simulink library "Kitchen_Lib"  (R2023a)
settings: Solver=VariableStepAuto  StartTime=0.0  StopTime=10.0  RelTol=1e-3  EnableMultiTasking=on
undefined symbols (not defined in the file): Kitc_BusTyp_P, Kitc_BusTypSkyr_C, Kitc_ColrLedColrls_C, Kitc_ColrLedGrn_C, Kitc_ColrLedRed_C, Kitc_ColrLedYlw_C, Kitc_StDgnWtrTank_C, Kitc_StElecPlugScktOffByClmp50_P, Kitc_StsDlyBlink_C, Kitc_StsErrBlink_C, Kitc_StsFctAcvn_P, Kitc_StsInfoBlink_C, Kitc_StsKitchnOffAutoIgOff_P, Kitc_StsKitchnOffBySwt_P, Kitc_StsKitchnOffDoorLockd_P, Kitc_StsKitchnOffIgOff_P, Kitc_StsKitchnOffUv_P, Kitc_StsKitchnOnBySwt_P, Kitc_StsKitchnOnNVM_P, Kitc_StsLedOff_C, Kitc_StsLedOn_C, Kitc_StsLrgCnsAcv_P, Kitc_StTrfrAnSwtInstd_P, Kitc_StTrfrSwtInstd_P, Kitc_TiKitcRefgtrOffDly_P, Kitc_ULowrThdBat_C, Kitc_UUpprThdBat_C, Kitc_ValFalse_C, Kitc_ValPwmFreq2_C, Kitc_ValPwmFreq_C, Kitc_ValTrue_C
libraries: MAN_Library x50, E2E_Lib x3
(part 7 of 13)

== system Kitchen_Lib/Kitchen/100ms/Kitchn/Subsystem1/Subsystem19/WaterTankEmptyDiagnostic/Diagno sticsDebouncing ==
  Error : Inport
  StartLock : Inport  Port=2
  IgnitionStatus : Inport  Port=3
  OnDelay : Inport  Port=4
  OffDelay : Inport  Port=5
  Constant1 : Constant  Value=uint32(100)  OutDataTypeStr=uint32
  Constant10 : Constant  Value=uint32(CycleTime)  OutDataTypeStr=uint32
  Constant11 : Constant  Value=uint32(1)  OutDataTypeStr=uint32
  Constant12 : Constant  Value=uint32(10)  OutDataTypeStr=uint32
  Constant13 : Constant  Value=uint32(100)  OutDataTypeStr=uint32
  Constant14 : Constant  Value=uint32(1000)  OutDataTypeStr=uint32
  DiagnosticsDebouncingOriginal : Subsystem  AncestorBlock=MAN_Library/BasicLibrary/DiagnosticsDebouncingOriginal
  Multiport Switch2 : MultiPortSwitch  Inputs=4  SaturateOnIntegerOverflow=off  InputSameDT=off
  Terminator : Terminator
  DiagnosticFlag : Outport
  wires:
  IgnitionStatus/1 -> DiagnosticsDebouncingOriginal/3(IgnitionStatus)
  OnDelay/1 -> DiagnosticsDebouncingOriginal/4(OnDelay)
  StartLock/1 -> DiagnosticsDebouncingOriginal/2(StartLock)
  OffDelay/1 -> DiagnosticsDebouncingOriginal/5(OffDelay)
  DiagnosticsDebouncingOriginal/1(DiagnosticFlag) -> DiagnosticFlag/1
  Error/1 -> DiagnosticsDebouncingOriginal/1(Error)
  Constant11/1 -> Multiport Switch2/2
  Constant12/1 -> Multiport Switch2/3
  Constant14/1 -> Multiport Switch2/5
  Constant13/1 -> Multiport Switch2/4
  Constant10/1 -> Multiport Switch2/1
  Multiport Switch2/1 -> Terminator/1
  Constant1/1 -> DiagnosticsDebouncingOriginal/6(CycleTime)

== system Kitchen_Lib/Kitchen/100ms/Kitchn/Subsystem1/Subsystem19/WaterTankEmptyDiagnostic/TurnOffDelay ==
  TurnOffDelayEnable : Inport
  TurnOffDelayThreshold : Inport  Port=2
  Constant1 : Constant  Value=uint32(100)  OutDataTypeStr=uint32
  Constant10 : Constant  Value=uint32(CycleTime)  OutDataTypeStr=uint32
  Constant11 : Constant  Value=uint32(1)  OutDataTypeStr=uint32
  Constant12 : Constant  Value=uint32(10)  OutDataTypeStr=uint32
  Constant13 : Constant  Value=uint32(100)  OutDataTypeStr=uint32
  Constant14 : Constant  Value=uint32(1000)  OutDataTypeStr=uint32
  Multiport Switch2 : MultiPortSwitch  Inputs=4  SaturateOnIntegerOverflow=off  InputSameDT=off
  Terminator : Terminator
  TurnOffDelayOriginal : Subsystem  AncestorBlock=MAN_Library/BasicLibrary/TurnOffDelayOriginal
  TurnOffDelayFlag : Outport
  TurnOffDelayExpiredTime : Outport  Port=2
  wires:
  TurnOffDelayOriginal/2(TurnOffDelayExpiredTime) -> TurnOffDelayExpiredTime/1
  TurnOffDelayOriginal/1(TurnOffDelayFlag) -> TurnOffDelayFlag/1
  TurnOffDelayThreshold/1 -> TurnOffDelayOriginal/2(TurnOffDelayThreshold)
  TurnOffDelayEnable/1 -> TurnOffDelayOriginal/1(TurnOffDelayEnable)
  Constant11/1 -> Multiport Switch2/2
  Constant12/1 -> Multiport Switch2/3
  Constant14/1 -> Multiport Switch2/5
  Constant13/1 -> Multiport Switch2/4
  Constant10/1 -> Multiport Switch2/1
  Multiport Switch2/1 -> Terminator/1
  Constant1/1 -> TurnOffDelayOriginal/3(CycleTime)

== system Kitchen_Lib/Kitchen/100ms/Kitchn/Subsystem1/Subsystem16/001_KitchnCtl/001_HostessSideButton/001_HostessSideTopButton ==
  note: Parameter
      | G_78_PARA_Enable_KuecheBeif_S
      | is deleted
  note: Parameter G_78_PARA_Enable_KuecheBeif_S is deleted
  Kitc_StKitcHostsSideSwtUpprPart : Inport
  SwtLock : Inport  Port=2
  "GW_ModeExbn " : Inport  Port=3
  "GW_StUvTopPrio " : Inport  Port=4
  Kitchn_On : Inport  Port=5
  Constant1 : Constant  Value=Kitc_ValFalse_C
  Constant3 : Constant  Value=Kitc_ValFalse_C
  Logical Operator{10,12,24..27} (6 alike) : Logic  Operator=NOT  Inputs=4  AllPortsSameDT=off  OutDataTypeStr=boolean
  Logical Operator11 : Logic  Operator=OR  Inputs=3  AllPortsSameDT=off  OutDataTypeStr=boolean
  Logical Operator23 : Logic  Inputs=6  AllPortsSameDT=off  OutDataTypeStr=boolean
  Logical Operator9 : Logic  Inputs=3  AllPortsSameDT=off  OutDataTypeStr=boolean
  RisingEdgeDetection : MAN_Library/RisingEdgeDetection
  HostessSideTopButtonErr : Outport
  HostessSideBottomButton_ON : Outport  Port=2
  wires:
  Kitc_StKitcHostsSideSwtUpprPart/1 -> RisingEdgeDetection/1
  Logical Operator25/1 -> Logical Operator23/3
  "GW_StUvTopPrio "/1 -> Logical Operator11/3, Logical Operator25/1
  Logical Operator24/1 -> Logical Operator23/2
  Logical Operator23/1 -> HostessSideBottomButton_ON/1
  Logical Operator9/1 -> HostessSideTopButtonErr/1
  SwtLock/1 -> Logical Operator11/2, Logical Operator26/1
  Logical Operator11/1 -> Logical Operator9/1
  Logical Operator12/1 -> Logical Operator11/1
  Logical Operator27/1 -> Logical Operator23/5
  "GW_ModeExbn "/1 -> Logical Operator10/1, Logical Operator24/1
  RisingEdgeDetection/1 -> Logical Operator23/1, Logical Operator9/3
  Kitchn_On/1 -> Logical Operator27/1
  Logical Operator26/1 -> Logical Operator23/4
  Constant1/1 -> Logical Operator12/1
  Constant3/1 -> Logical Operator23/6
  Logical Operator10/1 -> Logical Operator9/2

== system Kitchen_Lib/Kitchen/100ms/Kitchn/Subsystem1/Subsystem16/001_KitchnCtl/001_HostessSideButton/002_HostessSideBottomButton ==
  note: Parameter G_78_PARA_Enable_KuecheBeif_S is deleted
  note: Parameter G_78_PARA_Enable_KuecheBeif_S is deleted
  Kitchn_On : Inport
  "GW_ModeExbn " : Inport  Port=2
  Kitc_StKitcHostsSideSwtBotmPart : Inport  Port=3
  SwtLock : Inport  Port=4
  Constant1 : Constant  Value=Kitc_ValFalse_C
  Constant2 : Constant  Value=Kitc_ValFalse_C
  Logical Operator14 : Logic  Inputs=3  AllPortsSameDT=off  OutDataTypeStr=boolean
  Logical Operator15 : Logic  Operator=OR  AllPortsSameDT=off  OutDataTypeStr=boolean
  Logical Operator{16..17,29..30} (4 alike) : Logic  Operator=NOT  Inputs=4  AllPortsSameDT=off  OutDataTypeStr=boolean
  Logical Operator28 : Logic  Inputs=5  AllPortsSameDT=off  OutDataTypeStr=boolean
  RisingEdgeDetection : MAN_Library/RisingEdgeDetection
  HostessSideBottomButtonErr : Outport
  HostessSideBottomButton_OFF : Outport  Port=2
  wires:
  Kitchn_On/1 -> Logical Operator28/4
  Logical Operator15/1 -> Logical Operator14/1
  Kitc_StKitcHostsSideSwtBotmPart/1 -> RisingEdgeDetection/1
  Logical Operator14/1 -> HostessSideBottomButtonErr/1
  Logical Operator17/1 -> Logical Operator15/1
  "GW_ModeExbn "/1 -> Logical Operator29/1, Logical Operator16/1
  Constant1/1 -> Logical Operator28/5
  Logical Operator30/1 -> Logical Operator28/3
  SwtLock/1 -> Logical Operator30/1, Logical Operator15/2
  Logical Operator28/1 -> HostessSideBottomButton_OFF/1
  RisingEdgeDetection/1 -> Logical Operator28/1, Logical Operator14/3
  Constant2/1 -> Logical Operator17/1
  Logical Operator16/1 -> Logical Operator14/2
  Logical Operator29/1 -> Logical Operator28/2

== system Kitchen_Lib/Kitchen/100ms/Kitchn/Subsystem1/Subsystem16/001_KitchnCtl/002_FlipFlop/KSW-KitchenControl ==
  ABat_StAddlBatInstd : Inport
  GW_StEngRung : Inport  Port=2
  "GW_Ubat " : Inport  Port=3
  "GW_StClmp50Off3Sec " : Inport  Port=4
  CLS_StDoorLockdOutd : Inport  Port=5
  Kitc_StsHostsCallAcv : Inport  Port=6
  "GW_ModeExbn " : Inport  Port=7
  "GW_StUvTopPrio " : Inport  Port=8
  GW_StClmp15 : Inport  Port=9
  Kitchn_On : Inport  Port=10
  KSW_Battery : Subsystem
  KitchenControl : Subsystem
  LrgCns : Outport
  Kitc_WarnLrgCns : Outport  Port=2
  Kitc_StsKitcAcv : Outport  Port=3
  Kitchn_HostsCallOn : Outport  Port=4
  Kitc_StLrgCns : Outport  Port=5
  Kitc_StSmlCns : Outport  Port=6
  Kitc_StWtrPump : Outport  Port=7
  Kitc_StBuzRe : Outport  Port=8
  Kitc_StKitcLi : Outport  Port=9
  Kitc_StsPwmFreq : Outport  Port=10
  wires:
  KSW_Battery/3(LrgCns) -> LrgCns/1
  "GW_Ubat "/1 -> KSW_Battery/2("GW_Ubat ")
  "GW_StClmp50Off3Sec "/1 -> KSW_Battery/6("GW_StClmp50Off3Sec ")
  KSW_Battery/4(Kitc_WarnLrgCns) -> Kitc_WarnLrgCns/1
  KSW_Battery/5(Kitc_StBuzRe) -> Kitc_StBuzRe/1
  CLS_StDoorLockdOutd/1 -> KSW_Battery/7(CLS_StDoorLockdOutd)
  Kitchn_On/1 -> KitchenControl/1(Kitchn_On), KSW_Battery/1(Kitchn_On)
  "GW_ModeExbn "/1 -> [GW_ModeExbn]
  "GW_StUvTopPrio "/1 -> [GW_StUvTopPrio]
  GW_StClmp15/1 -> [GW_StClmp15]
  [GW_StClmp15] -> KSW_Battery/3(GW_StClmp15)
  [GW_StUvTopPrio] -> KSW_Battery/4("GW_StUvTopPrio ")
  [GW_ModeExbn] -> KSW_Battery/5("GW_ModeExbn ")
  Kitc_StsHostsCallAcv/1 -> KSW_Battery/8(Kitc_StsHostsCallAcv)
  KitchenControl/1(Kitc_StsKitcAcv) -> Kitc_StsKitcAcv/1
  KitchenControl/2(Kitchn_HostsCallOn) -> Kitchn_HostsCallOn/1
  KitchenControl/3(Kitc_StLrgCns) -> Kitc_StLrgCns/1
  ABat_StAddlBatInstd/1 -> KSW_Battery/10(ABat_StAddlBatInstd), KitchenControl/6(ABat_StAddlBatInstd)
  GW_StEngRung/1 -> KSW_Battery/9(GW_StEngRung), KitchenControl/7(GW_StEngRung)
  KSW_Battery/1(KitchnAcv) -> KitchenControl/2(KitchnAcv)
  [GW_ModeExbn] -> KitchenControl/4("GW_ModeExbn ")
  [GW_StClmp15] -> KitchenControl/5(GW_StClmp15)
  KitchenControl/5(Kitc_StWtrPump) -> Kitc_StWtrPump/1
  KitchenControl/6(Kitc_StKitcLi) -> Kitc_StKitcLi/1
  KitchenControl/4(Kitc_StSmlCns) -> Kitc_StSmlCns/1
  KSW_Battery/2(LrgCnsEna) -> KitchenControl/3(LrgCnsEna)
  KitchenControl/7(Kitc_StsPwmFreq) -> Kitc_StsPwmFreq/1

== system Kitchen_Lib/Kitchen/100ms/Kitchn/Subsystem1/Subsystem16/001_KitchnCtl/002_FlipFlop/KitchenEnable ==
  Kitc_StKitcSwtUpprPart : Inport
  HostsSideTopBtn_ON : Inport  Port=2
  HostsSideBotmBtn_OFF : Inport  Port=3
  Kitc_StKitcSwtBotmPart : Inport  Port=4
  CLS_StDoorLockdOutd : Inport  Port=5
  "GW_StStrtNew " : Inport  Port=6
  "GW_ModeExbn " : Inport  Port=7
  "GW_StUvTopPrio " : Inport  Port=8
  GW_StClmp15 : Inport  Port=9
  Kitc_StDemoBd : Inport  Port=10
  Kitc_TdOff : Inport  Port=11
  KitchenOffAutomaticIgnitionOff : Subsystem
  KitchenOffBySwitch : Subsystem
  KitchenOffDoorLocked : Subsystem
  KitchenOffIgnitionOff : Subsystem
  KitchenOffUndervoltage : Subsystem
  KitchenOnBySwitch : Subsystem
  KitchenOnNVM : Subsystem
  Logical Operator4 : Logic  Operator=OR  Inputs=9  AllPortsSameDT=off  OutDataTypeStr=boolean
  Subsystem : Subsystem
  Unit Delay : UnitDelay  SampleTime=-1  HasFrameUpgradeWarning=on
  Unit Delay1 : UnitDelay  SampleTime=-1  HasFrameUpgradeWarning=on
  Kitchn_On : Outport
  wires:
  HostsSideTopBtn_ON/1 -> Logical Operator4/9
  Subsystem/1(Kitchn_On) -> Unit Delay/1, Kitchn_On/1
  Logical Operator4/1 -> Subsystem/1(StateChange)
  "GW_ModeExbn "/1 -> [GW_ModeExbn]
  "GW_StUvTopPrio "/1 -> [GW_StUvTopPrio]
  GW_StClmp15/1 -> [GW_StClmp15]
  Unit Delay/1 -> [Kitchn_On]
  HostsSideBotmBtn_OFF/1 -> Logical Operator4/8, KitchenOnNVM/6(HostsSideBotmBtn_OFF)
  Kitc_StKitcSwtUpprPart/1 -> KitchenOnBySwitch/1(Kitc_StKitcSwtUpprPart)
  KitchenOnBySwitch/1("KitchnOnBySwt ") -> Logical Operator4/1
  Kitc_StKitcSwtBotmPart/1 -> KitchenOffBySwitch/1(Kitc_StKitcSwtBotmPart)
  KitchenOffBySwitch/1(KitchnOffBySwt) -> Logical Operator4/2, [KitchnOffBySwt]
  KitchenOffIgnitionOff/1(KitchnOffIgOff) -> Logical Operator4/3
  Kitc_StDemoBd/1 -> KitchenOffAutomaticIgnitionOff/1(Kitc_StDemoBd)
  Kitc_TdOff/1 -> KitchenOffAutomaticIgnitionOff/2(Kitc_TdOff)
  KitchenOffAutomaticIgnitionOff/1("KitchnOffAutoIgOff ") -> Logical Operator4/4
  CLS_StDoorLockdOutd/1 -> KitchenOffDoorLocked/1(CLS_StDoorLockdOutd)
  KitchenOffDoorLocked/1(KitchnOffDoorLockd) -> Logical Operator4/5
  KitchenOffUndervoltage/1(KitchnOffUv) -> Logical Operator4/6
  "GW_StStrtNew "/1 -> KitchenOnNVM/1("GW_StStrtNew ")
  KitchenOnNVM/1("KitchnOnNVM  ") -> Logical Operator4/7
  [Kitchn_On] -> KitchenOnBySwitch/4(Kitchn_On)
  [GW_ModeExbn] -> KitchenOnBySwitch/2("GW_ModeExbn ")
  [GW_StUvTopPrio] -> KitchenOnBySwitch/3("GW_StUvTopPrio ")
  [GW_StClmp15] -> KitchenOffIgnitionOff/1(GW_StClmp15)
  [Kitchn_On] -> KitchenOffIgnitionOff/2(Kitchen_On)
  [Kitchn_On] -> KitchenOffBySwitch/3(Kitchen_On)
  [GW_ModeExbn] -> KitchenOffBySwitch/2("GW_ModeExbn ")
  [GW_StClmp15] -> KitchenOffAutomaticIgnitionOff/3(GW_StClmp15)
  [Kitchn_On] -> KitchenOffAutomaticIgnitionOff/4(Kitchen_On)
  [GW_StClmp15] -> KitchenOffDoorLocked/2(GW_StClmp15)
  [Kitchn_On] -> KitchenOffDoorLocked/3(Kitchen_On)
  [Kitchn_On] -> KitchenOffUndervoltage/2(Kitchen_On)
  [GW_StUvTopPrio] -> KitchenOffUndervoltage/1("GW_StUvTopPrio ")
  [GW_StClmp15] -> KitchenOnNVM/3(GW_StClmp15)
  [Kitchn_On] -> KitchenOnNVM/4(Kitchen_On)
  [GW_ModeExbn] -> KitchenOnNVM/2("GW_ModeExbn ")
  [KitchnOffBySwt] -> Unit Delay1/1
  Unit Delay1/1 -> KitchenOnNVM/5(KitchnOffBySwt)

== system Kitchen_Lib/Kitchen/100ms/Kitchn/Subsystem1/Subsystem16/001_KitchnCtl/003_KitchenDriver/Diagnostic ==
  Kitc_StsWtrTankEmpty : Inport
  "GW_StrtLock " : Inport  Port=2
  "GW_StClmp15On3Sec " : Inport  Port=3
  "Constant                                         " : MAN_Library/TimeConstant  hours=0  minutes=0  seconds=3  miliseconds=0
  "Constant1                                        " : MAN_Library/TimeConstant  hours=0  minutes=0  seconds=30  miliseconds=0
  "Constant2                                        " : MAN_Library/TimeConstant  hours=0  minutes=1  seconds=0  miliseconds=0
  Constant8 : Constant  Value=Kitc_ValTrue_C
  DIAG : Subsystem
  Diagno sticsDebouncing : MAN_Library/DiagnosticsDebouncing  CycleTime=Cycle Time: 10 Ms
  Terminator : Terminator
  TurnOffDelay : MAN_Library/TurnOffDelay  CycleTime=Cycle Time: 10 Ms
  wires:
  "GW_StrtLock "/1 -> Diagno sticsDebouncing/2
  "GW_StClmp15On3Sec "/1 -> Diagno sticsDebouncing/3
  TurnOffDelay/1 -> Diagno sticsDebouncing/1
  "Constant                                         "/1 -> TurnOffDelay/2
  "Constant1                                        "/1 -> Diagno sticsDebouncing/4
  "Constant2                                        "/1 -> Diagno sticsDebouncing/5
  Kitc_StsWtrTankEmpty/1 -> TurnOffDelay/1
  TurnOffDelay/2 -> Terminator/1
  Diagno sticsDebouncing/1 -> DIAG/1(In1)
  Constant8/1 -> DIAG/2(In2)

== system Kitchen_Lib/Kitchen/100ms/Kitchn/Subsystem1/Subsystem16/001_KitchnCtl/004_Led/HostessError ==
  HostSideButtonLock : Inport
  Kitc_WarnLrgCns : Inport  Port=2
  Constant1 : Constant  Value=Kitc_BusTypSkyr_C
  Constant2 : Constant  Value=Kitc_BusTyp_P
  Logical Operator14 : Logic  AllPortsSameDT=off  OutDataTypeStr=boolean
  Logical Operator15 : Logic  Operator=NOT  Inputs=4  AllPortsSameDT=off  OutDataTypeStr=boolean
  Multiport Switch3 : MultiPortSwitch  DataPortOrder=Zero-based contiguous  Inputs=2  zeroidx=on  SaturateOnIntegerOverflow=off  InputSameDT=off
  Relational Operator1 : RelationalOperator  Operator===  OutDataTypeStr=boolean  InputSameDT=off
  HosstesErr : Outport
  wires:
  HostSideButtonLock/1 -> Multiport Switch3/3, Logical Operator14/2
  Relational Operator1/1 -> Multiport Switch3/1
  Multiport Switch3/1 -> HosstesErr/1
  Logical Operator14/1 -> Multiport Switch3/2
  Logical Operator15/1 -> Logical Operator14/1
  Kitc_WarnLrgCns/1 -> Logical Operator15/1
  Constant2/1 -> Relational Operator1/1
  Constant1/1 -> Relational Operator1/2

== system Kitchen_Lib/Kitchen/100ms/Kitchn/Subsystem1/Subsystem16/001_KitchnCtl/004_Led/HostessGreenDelay ==
  LrgCns : Inport
  Kitchn_On : Inport  Port=2
  Kitc_WarnLrgCns : Inport  Port=3
  HostSideButtonLock : Inport  Port=4
  HostsCallAcv : Inport  Port=5
  Constant10 : Constant  Value=Kitc_BusTypSkyr_C
  Constant12 : Constant  Value=Kitc_BusTyp_P
  Constant2 : Constant  Value=Kitc_ValFalse_C
  Data Type Conversion : DataTypeConversion  OutDataTypeStr=uint8  SaturateOnIntegerOverflow=off  RndMeth=Floor
  Logical Operator{8..11} (4 alike) : Logic  Operator=NOT  Inputs=4  AllPortsSameDT=off  OutDataTypeStr=boolean
  Logical Operator7 : Logic  Inputs=5  AllPortsSameDT=off  OutDataTypeStr=boolean
  Multiport Switch4 : MultiPortSwitch  DataPortOrder=Zero-based contiguous  Inputs=2  zeroidx=on  SaturateOnIntegerOverflow=off  InputSameDT=off
  Relational Operator : RelationalOperator  Operator===  OutDataTypeStr=boolean  InputSameDT=off
  HostessGreenDly : Outport
  wires:
  Constant10/1 -> Relational Operator/2
  Constant12/1 -> Relational Operator/1
  Relational Operator/1 -> Multiport Switch4/1
  Multiport Switch4/1 -> HostessGreenDly/1
  HostsCallAcv/1 -> Logical Operator10/1
  Kitchn_On/1 -> Logical Operator7/3
  Logical Operator8/1 -> Logical Operator7/5
  LrgCns/1 -> Logical Operator9/1
  Logical Operator9/1 -> Logical Operator7/2
  Logical Operator10/1 -> Logical Operator7/4
  Logical Operator11/1 -> Logical Operator7/1
  Kitc_WarnLrgCns/1 -> Logical Operator11/1
  Constant2/1 -> Data Type Conversion/1
  Data Type Conversion/1 -> Multiport Switch4/3
  Logical Operator7/1 -> Multiport Switch4/2
  HostSideButtonLock/1 -> Logical Operator8/1

== system Kitchen_Lib/Kitchen/100ms/Kitchn/Subsystem1/Subsystem16/001_KitchnCtl/004_Led/HostessGreenOn ==
  LrgCns : Inport
  Kitchn_On : Inport  Port=2
  Kitc_WarnLrgCns : Inport  Port=3
  HostSideButtonLock : Inport  Port=4
  HostsCallAcv : Inport  Port=5
  Constant10 : Constant  Value=Kitc_BusTypSkyr_C
  Constant12 : Constant  Value=Kitc_BusTyp_P
  Logical Operator1 : Logic  Inputs=4  AllPortsSameDT=off  OutDataTypeStr=boolean
  Logical Operator{2..5,54} (5 alike) : Logic  Operator=NOT  Inputs=4  AllPortsSameDT=off  OutDataTypeStr=boolean
  Logical Operator52 : Logic  Inputs=3  AllPortsSameDT=off  OutDataTypeStr=boolean
  Multiport Switch4 : MultiPortSwitch  DataPortOrder=Zero-based contiguous  Inputs=2  zeroidx=on  SaturateOnIntegerOverflow=off  InputSameDT=off
  Relational Operator : RelationalOperator  Operator===  OutDataTypeStr=boolean  InputSameDT=off
  HostessGreenOn : Outport
  wires:
  Multiport Switch4/1 -> HostessGreenOn/1
  Relational Operator/1 -> Multiport Switch4/1
  Constant12/1 -> Relational Operator/1
  Constant10/1 -> Relational Operator/2
  HostsCallAcv/1 -> Logical Operator54/1, Logical Operator3/1
  Kitchn_On/1 -> Logical Operator52/1
  Logical Operator52/1 -> Multiport Switch4/3
  Logical Operator54/1 -> Logical Operator52/3
  HostSideButtonLock/1 -> Logical Operator5/1, Logical Operator4/1
  Logical Operator1/1 -> Multiport Switch4/2
  LrgCns/1 -> Logical Operator1/1
  Logical Operator2/1 -> Logical Operator1/2
  Logical Operator3/1 -> Logical Operator1/3
  Kitc_WarnLrgCns/1 -> Logical Operator2/1
  Logical Operator4/1 -> Logical Operator1/4
  Logical Operator5/1 -> Logical Operator52/2

== system Kitchen_Lib/Kitchen/100ms/Kitchn/Subsystem1/Subsystem16/001_KitchnCtl/004_Led/HostessRed ==
  Kitc_WarnLrgCns : Inport
  HostSideButtonLock : Inport  Port=2
  HostsCallAcv : Inport  Port=3
  Constant10 : Constant  Value=Kitc_BusTypSkyr_C
  Constant12 : Constant  Value=Kitc_BusTyp_P
  Logical Operator12 : Logic  AllPortsSameDT=off  OutDataTypeStr=boolean
  Logical Operator13 : Logic  Operator=NOT  Inputs=4  AllPortsSameDT=off  OutDataTypeStr=boolean
  Logical Operator5 : Logic  AllPortsSameDT=off  OutDataTypeStr=boolean
  Logical Operator8 : Logic  Operator=NOT  Inputs=4  AllPortsSameDT=off  OutDataTypeStr=boolean
  Multiport Switch4 : MultiPortSwitch  DataPortOrder=Zero-based contiguous  Inputs=2  zeroidx=on  SaturateOnIntegerOverflow=off  InputSameDT=off
  Relational Operator : RelationalOperator  Operator===  OutDataTypeStr=boolean  InputSameDT=off
  HostessRed : Outport
  wires:
  Multiport Switch4/1 -> HostessRed/1
  Relational Operator/1 -> Multiport Switch4/1
  Constant12/1 -> Relational Operator/1
  Constant10/1 -> Relational Operator/2
  Logical Operator5/1 -> Multiport Switch4/3, Logical Operator12/2
  HostsCallAcv/1 -> Logical Operator5/1
  Logical Operator8/1 -> Logical Operator5/2
  Logical Operator12/1 -> Multiport Switch4/2
  Logical Operator13/1 -> Logical Operator12/1
  Kitc_WarnLrgCns/1 -> Logical Operator13/1
  HostSideButtonLock/1 -> Logical Operator8/1

== system Kitchen_Lib/Kitchen/100ms/Kitchn/Subsystem1/Subsystem16/001_KitchnCtl/004_Led/KitchenError ==
  note: TFoE
  "GW_ModeExbn " : Inport
  "GW_StUvTopPrio " : Inport  Port=2
  In3 : Inport  Port=3
  Kitc_StKitcSwtUpprPart : Inport  Port=4
  Kitc_WarnLrgCns : Inport  Port=5
  Constant1 : Constant  Value=Kitc_BusTypSkyr_C
  Constant2 : Constant  Value=Kitc_BusTyp_P
  Logical Operator21 : Logic  Operator=NOT  Inputs=4  AllPortsSameDT=off  OutDataTypeStr=boolean
  Logical Operator22 : Logic  AllPortsSameDT=off  OutDataTypeStr=boolean
  Logical Operator23 : Logic  Operator=NOT  Inputs=4  AllPortsSameDT=off  OutDataTypeStr=boolean
  Logical Operator4 : Logic  Inputs=3  AllPortsSameDT=off  OutDataTypeStr=boolean
  Multiport Switch6 : MultiPortSwitch  DataPortOrder=Zero-based contiguous  Inputs=2  zeroidx=on  SaturateOnIntegerOverflow=off  InputSameDT=off
  Relational Operator1 : RelationalOperator  Operator===  OutDataTypeStr=boolean  InputSameDT=off
  RisingEdgeDetection : MAN_Library/RisingEdgeDetection
  Terminator3 : Terminator
  TurnOffDelay : MAN_Library/TurnOffDelay  CycleTime=Cycle Time: 10 Ms
  KitchenErr : Outport
  wires:
  In3/1 -> TurnOffDelay/2
  TurnOffDelay/1 -> Logical Operator22/2, Multiport Switch6/3
  Kitc_StKitcSwtUpprPart/1 -> RisingEdgeDetection/1
  "GW_StUvTopPrio "/1 -> Logical Operator4/2
  "GW_ModeExbn "/1 -> Logical Operator21/1
  Logical Operator4/1 -> TurnOffDelay/1
  RisingEdgeDetection/1 -> Logical Operator4/3
  Logical Operator21/1 -> Logical Operator4/1
  Multiport Switch6/1 -> KitchenErr/1
  Logical Operator23/1 -> Logical Operator22/1
  Logical Operator22/1 -> Multiport Switch6/2
  Kitc_WarnLrgCns/1 -> Logical Operator23/1
  Relational Operator1/1 -> Multiport Switch6/1
  TurnOffDelay/2 -> Terminator3/1
  Constant2/1 -> Relational Operator1/1
  Constant1/1 -> Relational Operator1/2

== system Kitchen_Lib/Kitchen/100ms/Kitchn/Subsystem1/Subsystem16/001_KitchnCtl/004_Led/KitchenGreenLed ==
  LrgCns : Inport
  Kitchn_On : Inport  Port=2
  Kitc_WarnLrgCns : Inport  Port=3
  Constant10 : Constant  Value=Kitc_BusTypSkyr_C
  Constant12 : Constant  Value=Kitc_BusTyp_P
  Logical Operator16 : Logic  AllPortsSameDT=off  OutDataTypeStr=boolean
  Logical Operator17 : Logic  Operator=NOT  Inputs=4  AllPortsSameDT=off  OutDataTypeStr=boolean
  Multiport Switch4 : MultiPortSwitch  DataPortOrder=Zero-based contiguous  Inputs=2  zeroidx=on  SaturateOnIntegerOverflow=off  InputSameDT=off
  Relational Operator : RelationalOperator  Operator===  OutDataTypeStr=boolean  InputSameDT=off
  KitchenGreenOn : Outport
  wires:
  Constant10/1 -> Relational Operator/2
  Constant12/1 -> Relational Operator/1
  Kitchn_On/1 -> Multiport Switch4/3
  LrgCns/1 -> Logical Operator16/1
  Relational Operator/1 -> Multiport Switch4/1
  Logical Operator16/1 -> Multiport Switch4/2
  Logical Operator17/1 -> Logical Operator16/2
  Kitc_WarnLrgCns/1 -> Logical Operator17/1
  Multiport Switch4/1 -> KitchenGreenOn/1

== system Kitchen_Lib/Kitchen/100ms/Kitchn/Subsystem1/Subsystem16/001_KitchnCtl/004_Led/KitchenGreenLedDelay ==
  LrgCns : Inport
  Kitchn_On : Inport  Port=2
  Kitc_WarnLrgCns : Inport  Port=3
  Constant10 : Constant  Value=Kitc_BusTypSkyr_C
  Constant12 : Constant  Value=Kitc_BusTyp_P
  Constant7 : Constant  Value=Kitc_ValFalse_C
  Data Type Conversion1 : DataTypeConversion  OutDataTypeStr=uint8  SaturateOnIntegerOverflow=off  RndMeth=Floor
  Logical Operator18 : Logic  Inputs=3  AllPortsSameDT=off  OutDataTypeStr=boolean
  Logical Operator19 : Logic  Operator=NOT  Inputs=4  AllPortsSameDT=off  OutDataTypeStr=boolean
  Logical Operator20 : Logic  Operator=NOT  Inputs=4  AllPortsSameDT=off  OutDataTypeStr=boolean
  Multiport Switch4 : MultiPortSwitch  DataPortOrder=Zero-based contiguous  Inputs=2  zeroidx=on  SaturateOnIntegerOverflow=off  InputSameDT=off
  Relational Operator : RelationalOperator  Operator===  OutDataTypeStr=boolean  InputSameDT=off
  KitchenGreenDly : Outport
  wires:
  Constant10/1 -> Relational Operator/2
  Constant12/1 -> Relational Operator/1
  Relational Operator/1 -> Multiport Switch4/1
  Logical Operator18/1 -> Multiport Switch4/2
  Multiport Switch4/1 -> KitchenGreenDly/1
  Kitchn_On/1 -> Logical Operator18/1
  LrgCns/1 -> Logical Operator19/1
  Logical Operator19/1 -> Logical Operator18/3
  Logical Operator20/1 -> Logical Operator18/2
  Kitc_WarnLrgCns/1 -> Logical Operator20/1
  Constant7/1 -> Data Type Conversion1/1
  Data Type Conversion1/1 -> Multiport Switch4/3

== system Kitchen_Lib/Kitchen/100ms/Kitchn/Subsystem1/Subsystem16/001_KitchnCtl/004_Led/KitchenYellowLed ==
  Kitc_WarnLrgCns : Inport
  Constant10 : Constant  Value=Kitc_BusTypSkyr_C
  Constant11 : Constant  Value=Kitc_ValFalse_C
  Constant12 : Constant  Value=Kitc_BusTyp_P
  Data Type Conversion2 : DataTypeConversion  OutDataTypeStr=uint8  SaturateOnIntegerOverflow=off  RndMeth=Floor
  Multiport Switch7 : MultiPortSwitch  DataPortOrder=Zero-based contiguous  Inputs=2  zeroidx=on  SaturateOnIntegerOverflow=off  InputSameDT=off
  Relational Operator : RelationalOperator  Operator===  OutDataTypeStr=boolean  InputSameDT=off
  KitchenYellow : Outport
  wires:
  Relational Operator/1 -> Multiport Switch7/1
  Data Type Conversion2/1 -> Multiport Switch7/3
  Multiport Switch7/1 -> KitchenYellow/1
  Kitc_WarnLrgCns/1 -> Multiport Switch7/2
  Constant11/1 -> Data Type Conversion2/1
  Constant10/1 -> Relational Operator/2
  Constant12/1 -> Relational Operator/1

== system Kitchen_Lib/Kitchen/100ms/Kitchn/Subsystem1/Subsystem16/001_KitchnCtl/004_Led/LedColrSts ==
  KitchenYellow : Inport
  KitchenGreenOn : Inport  Port=2
  KitchenGreenDly : Inport  Port=3
  HostessGreenOn : Inport  Port=4
  HostessGreenDly : Inport  Port=5
  HosstesRed : Inport  Port=6
  HosstesErr : Inport  Port=7
  KitchenErr : Inport  Port=8
  Constant : Constant  Value=Kitc_ColrLedRed_C
  Constant1 : Constant  Value=Kitc_ColrLedYlw_C
  Constant10 : Constant  Value=Kitc_ColrLedYlw_C
  Constant11 : Constant  Value=Kitc_StsDlyBlink_C
  Constant12 : Constant  Value=Kitc_ColrLedColrls_C
  Constant13 : Constant  Value=Kitc_ColrLedGrn_C
  Constant{6,14..15,17} (4 alike) : Constant  Value=Kitc_StsErrBlink_C
  Constant16 : Constant  Value=Kitc_StsDlyBlink_C
  Constant18 : Constant  Value=Kitc_ColrLedColrls_C
  Constant2 : Constant  Value=Kitc_ColrLedGrn_C
  Constant3 : Constant  Value=Kitc_StsLedOff_C
  Constant4 : Constant  Value=Kitc_StsLedOn_C
  Constant5 : Constant  Value=Kitc_StsInfoBlink_C
  Constant7 : Constant  Value=Kitc_StsLedOff_C
  Constant8 : Constant  Value=Kitc_StsLedOn_C
  Constant9 : Constant  Value=Kitc_ColrLedRed_C
  Logical Operator : Logic  Operator=OR  AllPortsSameDT=off  OutDataTypeStr=boolean
  Logical Operator1 : Logic  Operator=OR  AllPortsSameDT=off  OutDataTypeStr=boolean
  Logical Operator2 : Logic  Operator=OR  AllPortsSameDT=off  OutDataTypeStr=boolean
  Multiport Switch{,1..14} (15 alike) : MultiPortSwitch  DataPortOrder=Zero-based contiguous  Inputs=2  zeroidx=on  SaturateOnIntegerOverflow=off  InputSameDT=off
  KitchenSwtLedColr : Outport
  KitchenSwtLedSts : Outport  Port=2
  KitchenHostessSideSwtLedColr : Outport  Port=3
  KitchenHostessSideSwtLedSts : Outport  Port=4
  wires:
  Multiport Switch/1 -> KitchenSwtLedColr/1
  Multiport Switch1/1 -> KitchenSwtLedSts/1
  Multiport Switch2/1 -> KitchenHostessSideSwtLedColr/1
  Constant/1 -> Multiport Switch/3
  Multiport Switch3/1 -> Multiport Switch/2
  Constant2/1 -> Multiport Switch14/3
  Constant1/1 -> Multiport Switch3/3
  KitchenGreenOn/1 -> Logical Operator/1, Multiport Switch6/1
  Multiport Switch4/1 -> Multiport Switch2/2
  HosstesRed/1 -> Multiport Switch9/1, Logical Operator2/1
  Constant9/1 -> Multiport Switch2/3
  Constant10/1 -> Multiport Switch4/3
  KitchenGreenDly/1 -> Logical Operator/2, Multiport Switch5/1
  Logical Operator/1 -> Multiport Switch14/1
  Constant6/1 -> Multiport Switch1/3
  Multiport Switch5/1 -> Multiport Switch13/2
  Constant11/1 -> Multiport Switch5/3
  Multiport Switch6/1 -> Multiport Switch5/2
  Constant4/1 -> Multiport Switch6/3
  Constant3/1 -> Multiport Switch6/2
  KitchenYellow/1 -> Multiport Switch3/1, Multiport Switch10/1, Multiport Switch4/1, Multiport Switch13/1
  Multiport Switch7/1 -> Multiport Switch4/2
  HostessGreenOn/1 -> Logical Operator1/1, Multiport Switch12/1
  HostessGreenDly/1 -> Logical Operator1/2, Multiport Switch11/1
  Logical Operator1/1 -> Multiport Switch7/1
  Constant12/1 -> Multiport Switch7/2
  Constant13/1 -> Multiport Switch7/3
  Multiport Switch8/1 -> KitchenHostessSideSwtLedSts/1
  Multiport Switch9/1 -> Multiport Switch8/2
  Constant14/1 -> Multiport Switch8/3
  Logical Operator2/1 -> Multiport Switch2/1
  HosstesErr/1 -> Logical Operator2/2, Multiport Switch8/1
  Constant5/1 -> Multiport Switch9/3
  Multiport Switch10/1 -> Multiport Switch9/2
  Constant15/1 -> Multiport Switch10/3
  Multiport Switch11/1 -> Multiport Switch10/2
  Constant16/1 -> Multiport Switch11/3
  Multiport Switch12/1 -> Multiport Switch11/2
  Constant7/1 -> Multiport Switch12/2
  Constant8/1 -> Multiport Switch12/3
  Multiport Switch13/1 -> Multiport Switch1/2
  Multiport Switch14/1 -> Multiport Switch3/2
  KitchenErr/1 -> Multiport Switch/1, Multiport Switch1/1
  Constant17/1 -> Multiport Switch13/3
  Constant18/1 -> Multiport Switch14/2

== system Kitchen_Lib/Kitchen/100ms/Kitchn/Subsystem1/Subsystem16/004_Trfr/002_FlipFlop/KSW-Nvm ==
  TurnOn : Inport
  TurnOff : Inport  Port=2
  "GW_StStrtNew " : Inport  Port=3
  Kitc_StTrfrWoutNewStrt : Inport  Port=4
  Data Store Write : DataStoreWrite  DataStoreName=Kitc_StsTurnOnByBtnNv  IndexOptions=Index vector (dialog)  Indices=1  OutputSizes=1
  Logical Operator : Logic  Operator=OR  AllPortsSameDT=off  OutDataTypeStr=boolean
  Logical Operator1 : Logic  Operator=NOT  AllPortsSameDT=off  OutDataTypeStr=boolean
  Logical Operator2 : Logic  AllPortsSameDT=off  OutDataTypeStr=boolean
  SR : MAN_Library/SR
  wires:
  TurnOn/1 -> SR/1
  Logical Operator/1 -> SR/2
  Kitc_StTrfrWoutNewStrt/1 -> Logical Operator1/1
  Logical Operator1/1 -> Logical Operator2/2
  "GW_StStrtNew "/1 -> Logical Operator2/1
  Logical Operator2/1 -> Logical Operator/2
  TurnOff/1 -> Logical Operator/1
  SR/1 -> Data Store Write/1

== system Kitchen_Lib/Kitchen/100ms/Kitchn/Subsystem1/Subsystem16/004_Trfr/002_FlipFlop/TurnOffByButton ==
  Kitc_StTrfrSwtLowrPart : Inport
  Kitc_StTrfrBotmBtm : Inport  Port=2
  Fnc_ON : Inport  Port=3
  Logical Operator11 : Logic  AllPortsSameDT=off  OutDataTypeStr=boolean
  Logical Operator9 : Logic  Operator=OR  AllPortsSameDT=off  OutDataTypeStr=boolean
  RisingEdgeDetection1 : MAN_Library/RisingEdgeDetection
  TurnOff : Outport
  wires:
  Kitc_StTrfrBotmBtm/1 -> Logical Operator9/2
  RisingEdgeDetection1/1 -> Logical Operator11/1
  Logical Operator9/1 -> RisingEdgeDetection1/1
  Fnc_ON/1 -> Logical Operator11/2
  Kitc_StTrfrSwtLowrPart/1 -> Logical Operator9/1
  Logical Operator11/1 -> TurnOff/1

== system Kitchen_Lib/Kitchen/100ms/Kitchn/Subsystem1/Subsystem16/004_Trfr/002_FlipFlop/TurnOffConditions ==
  GW_StEngRung : Inport
  ABat_StAddlBatInstd : Inport  Port=2
  GW_StClmp15 : Inport  Port=3
  "GW_StUvNormPrio " : Inport  Port=4
  Fnc_ON : Inport  Port=5
  FallingEdgeDetection : MAN_Library/FallingEdgeDetection
  FallingEdgeDetection1 : MAN_Library/FallingEdgeDetection
  Logical Operator13 : Logic  AllPortsSameDT=off  OutDataTypeStr=boolean
  Logical Operator14 : Logic  Operator=NOT  AllPortsSameDT=off  OutDataTypeStr=boolean
  Logical Operator15 : Logic  Operator=OR  Inputs=3  AllPortsSameDT=off  OutDataTypeStr=boolean
  Logical Operator16 : Logic  AllPortsSameDT=off  OutDataTypeStr=boolean
  RisingEdgeDetection2 : MAN_Library/RisingEdgeDetection
  CdnOff : Outport
  wires:
  "GW_StUvNormPrio "/1 -> RisingEdgeDetection2/1
  Logical Operator14/1 -> Logical Operator16/2
  RisingEdgeDetection2/1 -> Logical Operator15/2
  GW_StEngRung/1 -> FallingEdgeDetection1/1
  Logical Operator15/1 -> Logical Operator13/2
  FallingEdgeDetection/1 -> Logical Operator15/1
  Fnc_ON/1 -> Logical Operator13/1
  FallingEdgeDetection1/1 -> Logical Operator16/1
  ABat_StAddlBatInstd/1 -> Logical Operator14/1
  Logical Operator16/1 -> Logical Operator15/3
  Logical Operator13/1 -> CdnOff/1
  GW_StClmp15/1 -> FallingEdgeDetection/1

== system Kitchen_Lib/Kitchen/100ms/Kitchn/Subsystem1/Subsystem16/004_Trfr/002_FlipFlop/TurnOnByButton ==
  Kitc_StTrfrSwtUpprPart : Inport
  Kitc_StTrfrSwtTopBtn : Inport  Port=2
  GW_StEngRung : Inport  Port=3
  ABat_StAddlBatInstd : Inport  Port=4
  GW_StClmp15 : Inport  Port=5
  "GW_StUvNormPrio " : Inport  Port=6
  Fnc_ON : Inport  Port=7
  Logical Operator10 : Logic  Operator=NOT  AllPortsSameDT=off  OutDataTypeStr=boolean
  Logical Operator12 : Logic  Operator=OR  AllPortsSameDT=off  OutDataTypeStr=boolean
  Logical Operator6 : Logic  Inputs=5  AllPortsSameDT=off  OutDataTypeStr=boolean
  Logical Operator7 : Logic  Operator=NOT  AllPortsSameDT=off  OutDataTypeStr=boolean
  Logical Operator8 : Logic  Operator=OR  AllPortsSameDT=off  OutDataTypeStr=boolean
  RisingEdgeDetection : MAN_Library/RisingEdgeDetection
  TurnOn : Outport
  wires:
  RisingEdgeDetection/1 -> Logical Operator6/5
  Logical Operator10/1 -> Logical Operator6/3
  Logical Operator12/1 -> Logical Operator6/1
  Fnc_ON/1 -> Logical Operator7/1
  Kitc_StTrfrSwtUpprPart/1 -> Logical Operator8/1
  ABat_StAddlBatInstd/1 -> Logical Operator12/2
  "GW_StUvNormPrio "/1 -> Logical Operator10/1
  Logical Operator7/1 -> Logical Operator6/4
  Kitc_StTrfrSwtTopBtn/1 -> Logical Operator8/2
  GW_StClmp15/1 -> Logical Operator6/2
  GW_StEngRung/1 -> Logical Operator12/1
  Logical Operator8/1 -> RisingEdgeDetection/1
  Logical Operator6/1 -> TurnOn/1

== system Kitchen_Lib/Kitchen/100ms/Kitchn/Subsystem1/Subsystem16/004_Trfr/002_FlipFlop/TurnOnNvm ==
  TrfrSwt : Inport
  Kitc_StsTurnOnByBtnNv : Inport  Port=2
  GW_StEngRung : Inport  Port=3
  ABat_StAddlBatInstd : Inport  Port=4
  GW_StClmp15 : Inport  Port=5
  Fnc_ON : Inport  Port=6
  GW_StUvNormPrio : Inport  Port=7
  Kitc_StsTurnOnByBtnNv1 : DataStoreWrite  DataStoreName=Kitc_StsTurnOnByBtnNv  IndexOptions=Index vector (dialog)  Indices=1  OutputSizes=1
  Logical Operator17 : Logic  Inputs=5  AllPortsSameDT=off  OutDataTypeStr=boolean
  Logical Operator18 : Logic  Operator=NOT  AllPortsSameDT=off  OutDataTypeStr=boolean
  Logical Operator19 : Logic  Operator=NOT  AllPortsSameDT=off  OutDataTypeStr=boolean
  Logical Operator20 : Logic  AllPortsSameDT=off  OutDataTypeStr=boolean
  Logical Operator21 : Logic  Operator=OR  AllPortsSameDT=off  OutDataTypeStr=boolean
  RisingEdgeDetection3 : MAN_Library/RisingEdgeDetection
  RisingEdgeDetection4 : MAN_Library/RisingEdgeDetection
  TurnOnNvm : Outport
  wires:
  Kitc_StsTurnOnByBtnNv/1 -> Logical Operator17/4
  Logical Operator20/1 -> Logical Operator21/2
  Fnc_ON/1 -> Logical Operator18/1
  RisingEdgeDetection3/1 -> Logical Operator21/1
  ABat_StAddlBatInstd/1 -> Logical Operator20/2
  Logical Operator19/1 -> Logical Operator17/3
  GW_StUvNormPrio/1 -> Logical Operator19/1
  Logical Operator18/1 -> Logical Operator17/2
  RisingEdgeDetection4/1 -> Logical Operator20/1
  Logical Operator21/1 -> Logical Operator17/5
  GW_StClmp15/1 -> RisingEdgeDetection4/1
  TrfrSwt/1 -> Logical Operator17/1
  Logical Operator17/1 -> Kitc_StsTurnOnByBtnNv1/1, TurnOnNvm/1
  GW_StEngRung/1 -> RisingEdgeDetection3/1

== system Kitchen_Lib/Kitchen/100ms/Kitchn/Subsystem1/Subsystem19/Cluster_Message/Subsystem2/Not_Released ==
  Released_Button : Inport
  GW_StUvTopPrio : Inport  Port=2
  Kitc_StClusterKitchnReleased : Inport  Port=3
  Enable : EnablePort
  FallingEdgeDetection : MAN_Library/FallingEdgeDetection
  FallingEdgeDetection1 : MAN_Library/FallingEdgeDetection
  Logical Operator : Logic  Operator=OR  AllPortsSameDT=off  OutDataTypeStr=boolean
  Logical Operator2 : Logic  AllPortsSameDT=off  OutDataTypeStr=boolean
  Logical Operator3 : Logic  AllPortsSameDT=off  OutDataTypeStr=boolean
  RisingEdgeDetection : MAN_Library/RisingEdgeDetection
  RisingEdgeDetection1 : MAN_Library/RisingEdgeDetection
  Kitc_StClusterNotReleased : Outport
  Kitc_StClusterLowBtNotReleased : Outport  Port=2
  wires:
  Logical Operator/1 -> Logical Operator3/2
  Logical Operator2/1 -> Kitc_StClusterNotReleased/1
  RisingEdgeDetection1/1 -> Logical Operator2/1
  FallingEdgeDetection1/1 -> Logical Operator2/2
  [Kitc_StClusterKitchnReleased] -> FallingEdgeDetection1/1
  FallingEdgeDetection/1 -> Logical Operator/1
  [Kitc_StClusterKitchnReleased] -> FallingEdgeDetection/1
  Kitc_StClusterKitchnReleased/1 -> [Kitc_StClusterKitchnReleased]
  GW_StUvTopPrio/1 -> [GW_StUvTopPrio]
  Logical Operator3/1 -> Kitc_StClusterLowBtNotReleased/1
  RisingEdgeDetection/1 -> Logical Operator/2
  Released_Button/1 -> [Kitc_StKitcSwtUpprPart]
  [Kitc_StKitcSwtUpprPart] -> RisingEdgeDetection/1
  [GW_StUvTopPrio] -> Logical Operator3/1
  [Kitc_StKitcSwtUpprPart] -> RisingEdgeDetection1/1

== system Kitchen_Lib/Kitchen/100ms/Kitchn/Subsystem1/Subsystem19/Cluster_Message/Subsystem2/Released ==
  Released_Button : Inport
  Enable : EnablePort
  Data Type Conversion : DataTypeConversion  OutDataTypeStr=boolean  SaturateOnIntegerOverflow=off  RndMeth=Floor
  RisingEdgeDetection : MAN_Library/RisingEdgeDetection
  Kitc_StClusterKitchnReleased : Outport
  wires:
  RisingEdgeDetection/1 -> Data Type Conversion/1
  Data Type Conversion/1 -> Kitc_StClusterKitchnReleased/1
  Released_Button/1 -> RisingEdgeDetection/1

== system Kitchen_Lib/Kitchen/100ms/Kitchn/Subsystem1/Subsystem19/Cluster_Message/Subsystem2/Subsystem ==
  GW_StUvTopPrio : Inport
  Kitc_StKitcSwtUpprPart : Inport  Port=2
  Logical Operator : Logic  AllPortsSameDT=off  OutDataTypeStr=boolean
  Logical Operator1 : Logic  Operator=NOT  AllPortsSameDT=off  OutDataTypeStr=boolean
  Out1 : Outport
  wires:
  GW_StUvTopPrio/1 -> Logical Operator1/1
  Kitc_StKitcSwtUpprPart/1 -> Logical Operator/2
  Logical Operator/1 -> Out1/1
  Logical Operator1/1 -> Logical Operator/1

== system Kitchen_Lib/Kitchen/100ms/Kitchn/Subsystem1/Subsystem19/Cluster_Message/Subsystem2/Subsystem1 ==
  Kitc_StClusterKitchnReleased : Inport
  GW_StUvTopPrio : Inport  Port=2
  Kitc_StKitcSwtUpprPart : Inport  Port=3
  GW_StClmp15 : Inport  Port=4
  SleepMode : Inport  Port=5
  FallingEdgeDetection : MAN_Library/FallingEdgeDetection
  Logical Operator : Logic  AllPortsSameDT=off  OutDataTypeStr=boolean
  Logical Operator1 : Logic  Operator=NOT  AllPortsSameDT=off  OutDataTypeStr=boolean
  Logical Operator2 : Logic  Operator=OR  Inputs=3  AllPortsSameDT=off  OutDataTypeStr=boolean
  Logical Operator3 : Logic  Operator=OR  Inputs=3  AllPortsSameDT=off  OutDataTypeStr=boolean
  Logical Operator4 : Logic  Operator=OR  AllPortsSameDT=off  OutDataTypeStr=boolean
  RisingEdgeDetection : MAN_Library/RisingEdgeDetection
  NotReleasedCondition : Outport
  wires:
  Logical Operator4/1 -> Logical Operator3/3
  FallingEdgeDetection/1 -> Logical Operator4/2
  RisingEdgeDetection/1 -> Logical Operator4/1
  GW_StClmp15/1 -> RisingEdgeDetection/1, FallingEdgeDetection/1
  Logical Operator3/1 -> NotReleasedCondition/1
  Logical Operator/1 -> Logical Operator3/2
  Logical Operator2/1 -> Logical Operator3/1
  SleepMode/1 -> Logical Operator2/1
  Kitc_StClusterKitchnReleased/1 -> Logical Operator2/2
  Logical Operator1/1 -> Logical Operator/1
  Kitc_StKitcSwtUpprPart/1 -> Logical Operator/2
  GW_StUvTopPrio/1 -> Logical Operator1/1, Logical Operator2/3

== system Kitchen_Lib/Kitchen/100ms/Kitchn/Subsystem1/Subsystem19/KSW_Battery/BatteryVoltageUnder23V/Constant3   ==
  Constant11 : Constant  Value=uint32(hours)  OutDataTypeStr=uint32
  Constant12 : Constant  Value=uint32(minutes)  OutDataTypeStr=uint32
  Constant13 : Constant  Value=uint32(miliseconds)  OutDataTypeStr=uint32
  Constant14 : Constant  Value=uint32(60)  OutDataTypeStr=uint32
  Constant15 : Constant  Value=uint32(1000)  OutDataTypeStr=uint32
  Constant16 : Constant  Value=uint32(seconds)  OutDataTypeStr=uint32
  Constant17 : Constant  Value=uint32(1000)  OutDataTypeStr=uint32
  Constant7 : Constant  Value=uint32(60)  OutDataTypeStr=uint32
  Constant8 : Constant  Value=uint32(60)  OutDataTypeStr=uint32
  Constant9 : Constant  Value=uint32(1000)  OutDataTypeStr=uint32
  Data Type Conversion{1..2,4..8,13..19} (14 alike) : DataTypeConversion  OutDataTypeStr=uint32  SaturateOnIntegerOverflow=off  RndMeth=Floor
  Product1 : Product  Inputs=4  OutDataTypeStr=uint32
  Product2 : Product  Inputs=3  OutDataTypeStr=uint32
  Product4 : Product  OutDataTypeStr=uint32
  Sum1 : Sum  Inputs=++++  AccumDataTypeStr=uint32
  time : Outport
  wires:
  Sum1/1 -> Data Type Conversion5/1  "time"
  Data Type Conversion5/1 -> time/1
  Constant7/1 -> Data Type Conversion13/1
  Data Type Conversion13/1 -> Product1/1
  Constant8/1 -> Data Type Conversion14/1
  Data Type Conversion14/1 -> Product1/2
  Constant9/1 -> Data Type Conversion15/1
  Data Type Conversion15/1 -> Product1/3
  Constant11/1 -> Data Type Conversion16/1
  Data Type Conversion16/1 -> Product1/4
  Constant12/1 -> Data Type Conversion2/1
  Constant14/1 -> Data Type Conversion17/1
  Data Type Conversion17/1 -> Product2/1
  Constant15/1 -> Data Type Conversion18/1
  Data Type Conversion18/1 -> Product2/2
  Constant17/1 -> Data Type Conversion19/1
  Data Type Conversion19/1 -> Product4/1
  Constant16/1 -> Data Type Conversion1/1
  Product1/1 -> Data Type Conversion4/1
  Product2/1 -> Data Type Conversion6/1
  Product4/1 -> Data Type Conversion7/1
  Data Type Conversion1/1 -> Product4/2
  Data Type Conversion2/1 -> Product2/3
  Constant13/1 -> Data Type Conversion8/1
  Data Type Conversion4/1 -> Sum1/1
  Data Type Conversion6/1 -> Sum1/2
  Data Type Conversion7/1 -> Sum1/3
  Data Type Conversion8/1 -> Sum1/4

== system Kitchen_Lib/Kitchen/100ms/Kitchn/Subsystem1/Subsystem19/KSW_Battery/BatteryVoltageUnder23V/Constant4   ==
  Constant11 : Constant  Value=uint32(hours)  OutDataTypeStr=uint32
  Constant12 : Constant  Value=uint32(minutes)  OutDataTypeStr=uint32
  Constant13 : Constant  Value=uint32(miliseconds)  OutDataTypeStr=uint32
  Constant14 : Constant  Value=uint32(60)  OutDataTypeStr=uint32
  Constant15 : Constant  Value=uint32(1000)  OutDataTypeStr=uint32
  Constant16 : Constant  Value=uint32(seconds)  OutDataTypeStr=uint32
  Constant17 : Constant  Value=uint32(1000)  OutDataTypeStr=uint32
  Constant7 : Constant  Value=uint32(60)  OutDataTypeStr=uint32
  Constant8 : Constant  Value=uint32(60)  OutDataTypeStr=uint32
  Constant9 : Constant  Value=uint32(1000)  OutDataTypeStr=uint32
  Data Type Conversion{1..2,4..8,13..19} (14 alike) : DataTypeConversion  OutDataTypeStr=uint32  SaturateOnIntegerOverflow=off  RndMeth=Floor
  Product1 : Product  Inputs=4  OutDataTypeStr=uint32
  Product2 : Product  Inputs=3  OutDataTypeStr=uint32
  Product4 : Product  OutDataTypeStr=uint32
  Sum1 : Sum  Inputs=++++  AccumDataTypeStr=uint32
  time : Outport
  wires:
  Sum1/1 -> Data Type Conversion5/1  "time"
  Data Type Conversion5/1 -> time/1
  Constant7/1 -> Data Type Conversion13/1
  Data Type Conversion13/1 -> Product1/1
  Constant8/1 -> Data Type Conversion14/1
  Data Type Conversion14/1 -> Product1/2
  Constant9/1 -> Data Type Conversion15/1
  Data Type Conversion15/1 -> Product1/3
  Constant11/1 -> Data Type Conversion16/1
  Data Type Conversion16/1 -> Product1/4
  Constant12/1 -> Data Type Conversion2/1
  Constant14/1 -> Data Type Conversion17/1
  Data Type Conversion17/1 -> Product2/1
  Constant15/1 -> Data Type Conversion18/1
  Data Type Conversion18/1 -> Product2/2
  Constant17/1 -> Data Type Conversion19/1
  Data Type Conversion19/1 -> Product4/1
  Constant16/1 -> Data Type Conversion1/1
  Product1/1 -> Data Type Conversion4/1
  Product2/1 -> Data Type Conversion6/1
  Product4/1 -> Data Type Conversion7/1
  Data Type Conversion1/1 -> Product4/2
  Data Type Conversion2/1 -> Product2/3
  Constant13/1 -> Data Type Conversion8/1
  Data Type Conversion4/1 -> Sum1/1
  Data Type Conversion6/1 -> Sum1/2
  Data Type Conversion7/1 -> Sum1/3
  Data Type Conversion8/1 -> Sum1/4

== system Kitchen_Lib/Kitchen/100ms/Kitchn/Subsystem1/Subsystem19/KSW_Battery/BatteryVoltageUnder23V/Constant6   ==
  Constant11 : Constant  Value=uint32(hours)  OutDataTypeStr=uint32
  Constant12 : Constant  Value=uint32(minutes)  OutDataTypeStr=uint32
  Constant13 : Constant  Value=uint32(miliseconds)  OutDataTypeStr=uint32
  Constant14 : Constant  Value=uint32(60)  OutDataTypeStr=uint32
  Constant15 : Constant  Value=uint32(1000)  OutDataTypeStr=uint32
  Constant16 : Constant  Value=uint32(seconds)  OutDataTypeStr=uint32
  Constant17 : Constant  Value=uint32(1000)  OutDataTypeStr=uint32
  Constant7 : Constant  Value=uint32(60)  OutDataTypeStr=uint32
  Constant8 : Constant  Value=uint32(60)  OutDataTypeStr=uint32
  Constant9 : Constant  Value=uint32(1000)  OutDataTypeStr=uint32
  Data Type Conversion{1..2,4..8,13..19} (14 alike) : DataTypeConversion  OutDataTypeStr=uint32  SaturateOnIntegerOverflow=off  RndMeth=Floor
  Product1 : Product  Inputs=4  OutDataTypeStr=uint32
  Product2 : Product  Inputs=3  OutDataTypeStr=uint32
  Product4 : Product  OutDataTypeStr=uint32
  Sum1 : Sum  Inputs=++++  AccumDataTypeStr=uint32
  time : Outport
  wires:
  Sum1/1 -> Data Type Conversion5/1  "time"
  Data Type Conversion5/1 -> time/1
  Constant7/1 -> Data Type Conversion13/1
  Data Type Conversion13/1 -> Product1/1
  Constant8/1 -> Data Type Conversion14/1
  Data Type Conversion14/1 -> Product1/2
  Constant9/1 -> Data Type Conversion15/1
  Data Type Conversion15/1 -> Product1/3
  Constant11/1 -> Data Type Conversion16/1
  Data Type Conversion16/1 -> Product1/4
  Constant12/1 -> Data Type Conversion2/1
  Constant14/1 -> Data Type Conversion17/1
  Data Type Conversion17/1 -> Product2/1
  Constant15/1 -> Data Type Conversion18/1
  Data Type Conversion18/1 -> Product2/2
  Constant17/1 -> Data Type Conversion19/1
  Data Type Conversion19/1 -> Product4/1
  Constant16/1 -> Data Type Conversion1/1
  Product1/1 -> Data Type Conversion4/1
  Product2/1 -> Data Type Conversion6/1
  Product4/1 -> Data Type Conversion7/1
  Data Type Conversion1/1 -> Product4/2
  Data Type Conversion2/1 -> Product2/3
  Constant13/1 -> Data Type Conversion8/1
  Data Type Conversion4/1 -> Sum1/1
  Data Type Conversion6/1 -> Sum1/2
  Data Type Conversion7/1 -> Sum1/3
  Data Type Conversion8/1 -> Sum1/4

== system Kitchen_Lib/Kitchen/100ms/Kitchn/Subsystem1/Subsystem19/KSW_Battery/BatteryVoltageUnder23V/TimePulse ==
  TimePulseEnable : Inport
  TimePulseDuration : Inport  Port=2
  Constant1 : Constant  Value=uint32(100)  OutDataTypeStr=uint32
  Constant10 : Constant  Value=uint32(CycleTime)  OutDataTypeStr=uint32
  Constant11 : Constant  Value=uint32(1)  OutDataTypeStr=uint32
  Constant12 : Constant  Value=uint32(10)  OutDataTypeStr=uint32
  Constant13 : Constant  Value=uint32(100)  OutDataTypeStr=uint32
  Constant14 : Constant  Value=uint32(1000)  OutDataTypeStr=uint32
  Multiport Switch2 : MultiPortSwitch  Inputs=4  SaturateOnIntegerOverflow=off  InputSameDT=off
  Terminator : Terminator
  TimePulseOriginal : Subsystem  AncestorBlock=MAN_Library/BasicLibrary/TimePulseOriginal
  TimePulseFlag : Outport
  TimePulseExpiredTime : Outport  Port=2
  wires:
  TimePulseOriginal/2(TimePulseExpiredTime) -> TimePulseExpiredTime/1
  TimePulseOriginal/1(TimePulseFlag) -> TimePulseFlag/1
  TimePulseEnable/1 -> TimePulseOriginal/1(TimePulseEnable)
  TimePulseDuration/1 -> TimePulseOriginal/2(TimePulseDuration)
  Constant11/1 -> Multiport Switch2/2
  Constant12/1 -> Multiport Switch2/3
  Constant14/1 -> Multiport Switch2/5
  Constant13/1 -> Multiport Switch2/4
  Constant10/1 -> Multiport Switch2/1
  Multiport Switch2/1 -> Terminator/1
  Constant1/1 -> TimePulseOriginal/3(CycleTime)

== system Kitchen_Lib/Kitchen/100ms/Kitchn/Subsystem1/Subsystem19/KSW_Battery/BatteryVoltageUnder23V/TimePulse1 ==
  TimePulseEnable : Inport
  TimePulseDuration : Inport  Port=2
  Constant1 : Constant  Value=uint32(100)  OutDataTypeStr=uint32
  Constant10 : Constant  Value=uint32(CycleTime)  OutDataTypeStr=uint32
  Constant11 : Constant  Value=uint32(1)  OutDataTypeStr=uint32
  Constant12 : Constant  Value=uint32(10)  OutDataTypeStr=uint32
  Constant13 : Constant  Value=uint32(100)  OutDataTypeStr=uint32
  Constant14 : Constant  Value=uint32(1000)  OutDataTypeStr=uint32
  Multiport Switch2 : MultiPortSwitch  Inputs=4  SaturateOnIntegerOverflow=off  InputSameDT=off
  Terminator : Terminator
  TimePulseOriginal : Subsystem  AncestorBlock=MAN_Library/BasicLibrary/TimePulseOriginal
  TimePulseFlag : Outport
  TimePulseExpiredTime : Outport  Port=2
  wires:
  TimePulseOriginal/2(TimePulseExpiredTime) -> TimePulseExpiredTime/1
  TimePulseOriginal/1(TimePulseFlag) -> TimePulseFlag/1
  TimePulseEnable/1 -> TimePulseOriginal/1(TimePulseEnable)
  TimePulseDuration/1 -> TimePulseOriginal/2(TimePulseDuration)
  Constant11/1 -> Multiport Switch2/2
  Constant12/1 -> Multiport Switch2/3
  Constant14/1 -> Multiport Switch2/5
  Constant13/1 -> Multiport Switch2/4
  Constant10/1 -> Multiport Switch2/1
  Multiport Switch2/1 -> Terminator/1
  Constant1/1 -> TimePulseOriginal/3(CycleTime)
